simulink model "SB13_stateflow_todo"  (R2024b)
settings: Solver=FixedStepDiscrete  StartTime=0.0  StopTime=30  FixedStep=0.05  RelTol=1e-3
undefined symbols (not defined in the file or in its folder): DiscIntNeverNeededParam
settings Model: Creator=admin  LastModifiedBy=admin

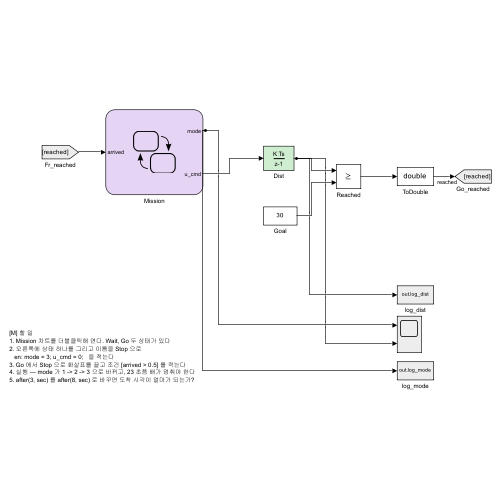
[thumbnail: Simulink's stored preview of the top-level diagram]
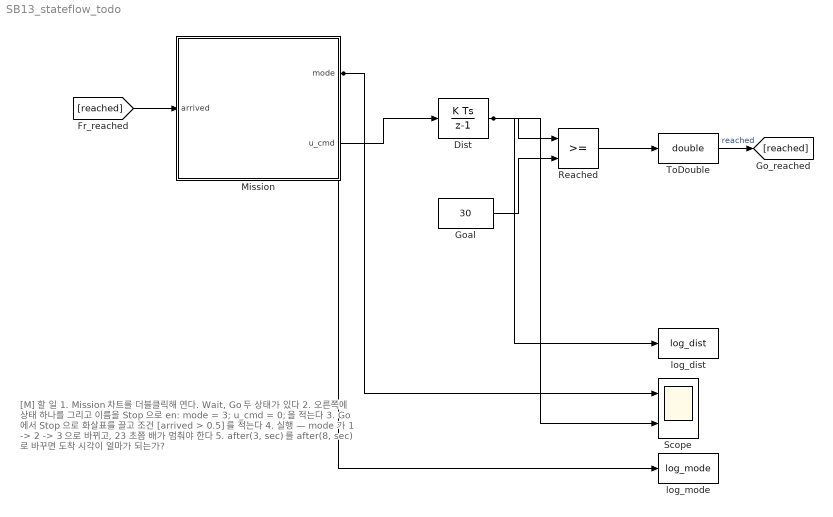
== system SB13_stateflow_todo ==
  note: [M] 할 일
      | 1. Mission 차트를 더블클릭해 연다. Wait, Go 두 상태가 있다
      | 2. 오른쪽에 상태 하나를 그리고 이름을 Stop 으로
      |    en: mode = 3; u_cmd = 0;   을 적는다
      | 3. Go 에서 Stop 으로 화살표를 끌고 조건 [arrived > 0.5] 를 적는다
      | 4. 실행 — mode 가 1 -> 2 -> 3 으로 바뀌고, 23 초쯤 배가 멈춰야 한다
      | 5. after(3, sec) 를 after(8, sec) 로 바꾸면 도착 시각이 얼마가 되는가?
  Dist : DiscreteIntegrator  SampleTime=0.05  ICPrevOutput=DiscIntNeverNeededParam  ICPrevScaledInput=DiscIntNeverNeededParam
  Goal : Constant  Value=30
  Mission : Stateflow chart  TreatAsAtomicUnit=on
  Reached : RelationalOperator  OutDataTypeStr=boolean  RndMeth=Simplest  InputSameDT=off
  Scope : Scope  NumInputPorts=2
  ToDouble : DataTypeConversion  OutDataTypeStr=double  SaturateOnIntegerOverflow=off  RndMeth=Floor
  log_dist : ToWorkspace  VariableName=log_dist  SaveFormat=Timeseries  SampleTime=0.05
  log_mode : ToWorkspace  VariableName=log_mode  SaveFormat=Timeseries  SampleTime=0.05
  wires:
  Mission/2(u_cmd) -> Dist/1
  Dist/1 -> Reached/1, log_dist/1, Scope/2
  Goal/1 -> Reached/2
  Reached/1 -> ToDouble/1
  ToDouble/1 -> [reached]  "reached"
  [reached] -> Mission/1(arrived)
  Mission/1(mode) -> log_mode/1, Scope/1

== stateflow chart SB13_stateflow_todo/Mission ==
  settings: updateMethod=DISCRETE  sampleTime=0.05
  state Wait
    en: mode = 1; u_cmd = 0;
  state Go
    en: mode = 2; u_cmd = 1.5;
  (default) -> Wait
  Wait -> Go : after(3, sec)
  data: arrived input; mode output; u_cmd output
